simulink model "omnirover3wd_multibody"  (R2026a)
settings: Solver=ode15s  StopTime=simulationStopTime  MaxStep=0.01
PreLoadFcn:
  | run(fullfile(fileparts(get_param(bdroot,'FileName')),'parameters.m'))
InitFcn:
  | addpath(fileparts(get_param(bdroot,'FileName')))
values from neighbouring files (symbols this model uses):
  chassisMass = roverMass - 3*(servoMass + wheelMass)    (= 0.18)    [parameters.m]
  commandVxWorld = 0.12    [parameters.m]
  commandVyWorld = 0.06    [parameters.m]
  commandYawRateWorld = 0.35    [parameters.m]
  floorDeflectionFilterTime = 2e-3    (= 0.002)    [parameters.m]
  floorLateralFriction = 0.0    (= 0)    [parameters.m]
  floorLongitudinalDynamicFriction = 0.65    [parameters.m]
  floorNominalDeflection = floorNominalLoadPerWheel/floorNormalStiffness    [parameters.m]
  floorNormalDamping = 450    [parameters.m]
  floorNormalStiffness = 1.5e5    (= 150000)    [parameters.m]
  servoMass = 0.055    [parameters.m]
  servoMaxSpeed = 62 * 2*pi / 60    (= 6.49262481742)    [parameters.m]
  wheelAngles = deg2rad([0 120 240])    [parameters.m]    (also in test_kinematics.m)
  wheelCenterRadius = roverDiameter/2 - wheelRadius    (= 0.056)    [parameters.m]    (also in test_kinematics.m)
  wheelForceLimit = servoMaxTorque / wheelRadius    (= 53.1193541667)    [parameters.m]
  wheelMass = 0.039    [parameters.m]
  wheelRadius = 0.024    [parameters.m]    (also in test_kinematics.m)
  wheelSpeedGain = -25    [parameters.m]
undefined symbols (not defined in the file or in its folder): omni3wdInverseKinematics, X, Y, Z
libraries: sm_lib x21, nesl_utility x19, sl_discontinuities x3
settings Model: Creator=cafdr  LastModifiedBy=cafdr

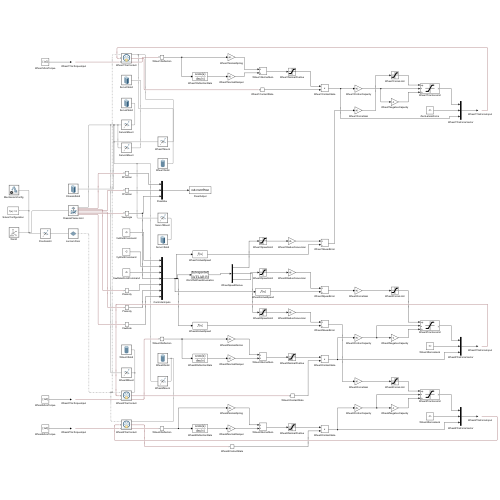
[thumbnail: Simulink's stored preview of the top-level diagram]
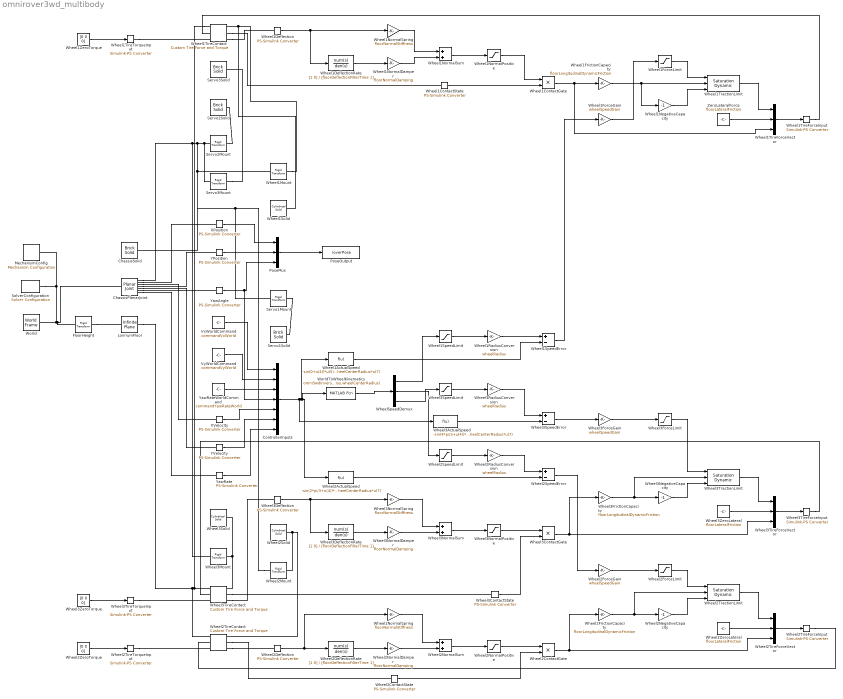
== system omnirover3wd_multibody ==
  ChassisPlanarJoint : sm_lib/Joints/Planar Joint  JointMode=Normal  CompositeWrenchDir=FollowerOnBase  CompositeWrenchFrame=BaseFrame  SenseConstraintForce=off  SenseConstraintTorque=off  SenseTotalForce=off  SenseTotalTorque=off  PxPositionTargetSpecify=off  PxPositionTargetPriority=High  PxPositionTargetValue=0  PxPositionTargetValueUnits=m  PxVelocityTargetSpecify=off  PxVelocityTargetPriority=High  PxVelocityTargetValue=0  PxVelocityTargetValueUnits=m/s  PxEquilibriumPosition=0  PxEquilibriumPositionUnits=m  PxSpringStiffness=0  PxSpringStiffnessUnits=N/m  PxDampingCoefficient=0  PxDampingCoefficientUnits=N/(m/s)  PxLowerLimitSpecify=off  PxLowerLimitBound=-1  PxLowerLimitBoundUnits=m  PxLowerLimitStiffness=1e6  PxLowerLimitStiffnessUnits=N/m  PxLowerLimitDamping=1e3  PxLowerLimitDampingUnits=N/(m/s)  PxLowerLimitTransitionRegionWidth=1e-4  PxLowerLimitTransitionRegionWidthUnits=m  PxUpperLimitSpecify=off  PxUpperLimitBound=1  PxUpperLimitBoundUnits=m  PxUpperLimitStiffness=1e6  PxUpperLimitStiffnessUnits=N/m  PxUpperLimitDamping=1e3  PxUpperLimitDampingUnits=N/(m/s)  PxUpperLimitTransitionRegionWidth=1e-4  PxUpperLimitTransitionRegionWidthUnits=m  PxTorqueActuationMode=NoTorque  PxMotionActuationMode=ComputedMotion  PxSensePosition=on  PxSenseVelocity=on  PxSenseAcceleration=off  PxSenseTorqueForce=off  PxSenseLowerLimitTorqueForce=off  PxSenseUpperLimitTorqueForce=off  PyPositionTargetSpecify=off  PyPositionTargetPriority=High  PyPositionTargetValue=0  PyPositionTargetValueUnits=m  PyVelocityTargetSpecify=off  PyVelocityTargetPriority=High  PyVelocityTargetValue=0  PyVelocityTargetValueUnits=m/s  PyEquilibriumPosition=0  PyEquilibriumPositionUnits=m  PySpringStiffness=0  PySpringStiffnessUnits=N/m  PyDampingCoefficient=0  PyDampingCoefficientUnits=N/(m/s)  PyLowerLimitSpecify=off  PyLowerLimitBound=-1  PyLowerLimitBoundUnits=m  PyLowerLimitStiffness=1e6  PyLowerLimitStiffnessUnits=N/m  PyLowerLimitDamping=1e3  PyLowerLimitDampingUnits=N/(m/s)  PyLowerLimitTransitionRegionWidth=1e-4  PyLowerLimitTransitionRegionWidthUnits=m  PyUpperLimitSpecify=off  PyUpperLimitBound=1  PyUpperLimitBoundUnits=m  PyUpperLimitStiffness=1e6  PyUpperLimitStiffnessUnits=N/m  PyUpperLimitDamping=1e3  PyUpperLimitDampingUnits=N/(m/s)  PyUpperLimitTransitionRegionWidth=1e-4  PyUpperLimitTransitionRegionWidthUnits=m  PyTorqueActuationMode=NoTorque  PyMotionActuationMode=ComputedMotion  PySensePosition=on  PySenseVelocity=on  PySenseAcceleration=off  PySenseTorqueForce=off  PySenseLowerLimitTorqueForce=off  PySenseUpperLimitTorqueForce=off  RzPositionTargetSpecify=off  RzPositionTargetPriority=High  RzPositionTargetValue=0  RzPositionTargetValueUnits=rad  RzVelocityTargetSpecify=off  RzVelocityTargetPriority=High  RzVelocityTargetValue=0  RzVelocityTargetValueUnits=rad/s  RzEquilibriumPosition=0  RzEquilibriumPositionUnits=deg  RzSpringStiffness=0  RzSpringStiffnessUnits=N*m/deg  RzDampingCoefficient=0  RzDampingCoefficientUnits=N*m/(deg/s)  RzLowerLimitSpecify=off  RzLowerLimitBound=-90  RzLowerLimitBoundUnits=deg  RzLowerLimitStiffness=1e4  RzLowerLimitStiffnessUnits=N*m/deg  RzLowerLimitDamping=10  RzLowerLimitDampingUnits=N*m/(deg/s)  RzLowerLimitTransitionRegionWidth=0.1  RzLowerLimitTransitionRegionWidthUnits=deg  RzUpperLimitSpecify=off  RzUpperLimitBound=90  RzUpperLimitBoundUnits=deg  RzUpperLimitStiffness=1e4  RzUpperLimitStiffnessUnits=N*m/deg  RzUpperLimitDamping=10  RzUpperLimitDampingUnits=N*m/(deg/s)  RzUpperLimitTransitionRegionWidth=0.1  RzUpperLimitTransitionRegionWidthUnits=deg  RzTorqueActuationMode=NoTorque  RzMotionActuationMode=ComputedMotion  RzSensePosition=on  RzSenseVelocity=on  RzSenseAcceleration=off  RzSenseTorqueForce=off  RzSenseLowerLimitTorqueForce=off  RzSenseUpperLimitTorqueForce=off
  ChassisSolid : sm_lib/Body Elements/Brick Solid  BrickDimensions=chassisDimensions  BrickDimensionsUnits=m  ExportEntireGeometry=off  InertiaType=CalculateFromGeometry  BasedOnType=Density  Density=1000  DensityUnits=kg/m^3  Mass=chassisMass  MassUnits=kg  CenterOfMass=[0 0 0]  CenterOfMassUnits=m  MomentsOfInertia=[1 1 1]  MomentsOfInertiaUnits=kg*m^2  ProductsOfInertia=[0 0 0]  ProductsOfInertiaUnits=kg*m^2  GraphicType=FromGeometry  MarkerShape=Sphere  MarkerSize=10  GraphicVisPropType=SimpleVisualProperties  GraphicDiffuseColor=[0.5 0.5 0.5]  GraphicOpacity=1  GraphicSpecularColor=[0.5 0.5 0.5 1.0]  GraphicAmbientColor=[0.15 0.15 0.15 1.0]  GraphicEmissiveColor=[0.0 0.0 0.0 1.0]  GraphicShininess=75  DoExposeReferenceFrame=on  SerializedFrames=<Frames/>
  ControllerInputs : Mux  Inputs=7
  FloorHeight : sm_lib/Frames and Transforms/Rigid Transform  RotationMethod=None  FollAlignAxisA=+X  BaseAlignAxisA=+Y  FollAlignAxisB=+Y  BaseAlignAxisB=+Z  RotationStandardAxis=+Z  RotationAngle=0  RotationAngleUnits=deg  RotationArbitraryAxis=[0 0 1]  RotationSequenceAxes=FollowerAxes  RotationSequence=XYX  RotationSequenceAngles=[0 0 0]  RotationSequenceAnglesUnits=deg  RotationMatrix=[1 0 0;0 1 0;0 0 1]  Quaternion=[1 0 0 0]  TranslationMethod=Cartesian  TranslationCartesianOffset=[0 0 -wheelRadius+floorNominalDeflection]  TranslationCartesianOffsetUnits=m  TranslationStandardAxis=+Z  TranslationStandardOffset=0  TranslationStandardOffsetUnits=m  TranslationROffset=0  TranslationROffsetUnits=m  TranslationThetaOffset=0  TranslationThetaOffsetUnits=deg  TranslationZOffset=0  TranslationZOffsetUnits=m
  LonriumFloor : sm_lib/Curves and Surfaces/Infinite Plane  GraphicType=Rectangle  GraphicPlaneWidth=2  GraphicPlaneWidthUnits=m  GraphicPlaneHeight=2  GraphicPlaneHeightUnits=m  GraphicVisPropType=SimpleVisualProperties  GraphicDiffuseColor=[0.55 0.58 0.62]  GraphicOpacity=1  GraphicSpecularColor=[0.5 0.5 0.5 1.0]  GraphicAmbientColor=[0.15 0.15 0.15 1.0]  GraphicEmissiveColor=[0.0 0.0 0.0 1.0]  GraphicShininess=75
  MechanismConfig : sm_lib/Utilities/Mechanism Configuration  UniformGravity=Constant  GravityVector=[0 0 -9.80665]  GravityVectorUnits=m/s^2  LinearizationDelta=0.001  JointModeTransitionNonlinearIterations=2
  PoseMux : Mux  Inputs=3
  PoseOutput : ToWorkspace  VariableName=roverPose  SaveFormat=Timeseries  SampleTime=-1
  Servo1Mount : sm_lib/Frames and Transforms/Rigid Transform  RotationMethod=RotationSequence  FollAlignAxisA=+X  BaseAlignAxisA=+Y  FollAlignAxisB=+Y  BaseAlignAxisB=+Z  RotationStandardAxis=+Z  RotationAngle=0  RotationAngleUnits=deg  RotationArbitraryAxis=[0 0 1]  RotationSequenceAxes=FollowerAxes  RotationSequence=ZYX  RotationSequenceAngles=[0 0 0]  RotationSequenceAnglesUnits=deg  RotationMatrix=[1 0 0;0 1 0;0 0 1]  Quaternion=[1 0 0 0]  TranslationMethod=Cartesian  TranslationCartesianOffset=(wheelCenterRadius-0.025)*[1 0 0]  TranslationCartesianOffsetUnits=m  TranslationStandardAxis=+Z  TranslationStandardOffset=0  TranslationStandardOffsetUnits=m  TranslationROffset=0  TranslationROffsetUnits=m  TranslationThetaOffset=0  TranslationThetaOffsetUnits=deg  TranslationZOffset=0  TranslationZOffsetUnits=m
  Servo1Solid : sm_lib/Body Elements/Brick Solid  BrickDimensions=servoDimensions  BrickDimensionsUnits=m  ExportEntireGeometry=off  InertiaType=CalculateFromGeometry  BasedOnType=Density  Density=1000  DensityUnits=kg/m^3  Mass=servoMass  MassUnits=kg  CenterOfMass=[0 0 0]  CenterOfMassUnits=m  MomentsOfInertia=[1 1 1]  MomentsOfInertiaUnits=kg*m^2  ProductsOfInertia=[0 0 0]  ProductsOfInertiaUnits=kg*m^2  GraphicType=FromGeometry  MarkerShape=Sphere  MarkerSize=10  GraphicVisPropType=SimpleVisualProperties  GraphicDiffuseColor=[0.5 0.5 0.5]  GraphicOpacity=1  GraphicSpecularColor=[0.5 0.5 0.5 1.0]  GraphicAmbientColor=[0.15 0.15 0.15 1.0]  GraphicEmissiveColor=[0.0 0.0 0.0 1.0]  GraphicShininess=75  DoExposeReferenceFrame=on  SerializedFrames=<Frames/>
  Servo2Mount : sm_lib/Frames and Transforms/Rigid Transform  RotationMethod=RotationSequence  FollAlignAxisA=+X  BaseAlignAxisA=+Y  FollAlignAxisB=+Y  BaseAlignAxisB=+Z  RotationStandardAxis=+Z  RotationAngle=0  RotationAngleUnits=deg  RotationArbitraryAxis=[0 0 1]  RotationSequenceAxes=FollowerAxes  RotationSequence=ZYX  RotationSequenceAngles=[120 0 0]  RotationSequenceAnglesUnits=deg  RotationMatrix=[1 0 0;0 1 0;0 0 1]  Quaternion=[1 0 0 0]  TranslationMethod=Cartesian  TranslationCartesianOffset=(wheelCenterRadius-0.025)*[cos(2*pi/3) sin(2*pi/3) 0]  TranslationCartesianOffsetUnits=m  TranslationStandardAxis=+Z  TranslationStandardOffset=0  TranslationStandardOffsetUnits=m  TranslationROffset=0  TranslationROffsetUnits=m  TranslationThetaOffset=0  TranslationThetaOffsetUnits=deg  TranslationZOffset=0  TranslationZOffsetUnits=m
  Servo2Solid : sm_lib/Body Elements/Brick Solid  BrickDimensions=servoDimensions  BrickDimensionsUnits=m  ExportEntireGeometry=off  InertiaType=CalculateFromGeometry  BasedOnType=Density  Density=1000  DensityUnits=kg/m^3  Mass=servoMass  MassUnits=kg  CenterOfMass=[0 0 0]  CenterOfMassUnits=m  MomentsOfInertia=[1 1 1]  MomentsOfInertiaUnits=kg*m^2  ProductsOfInertia=[0 0 0]  ProductsOfInertiaUnits=kg*m^2  GraphicType=FromGeometry  MarkerShape=Sphere  MarkerSize=10  GraphicVisPropType=SimpleVisualProperties  GraphicDiffuseColor=[0.5 0.5 0.5]  GraphicOpacity=1  GraphicSpecularColor=[0.5 0.5 0.5 1.0]  GraphicAmbientColor=[0.15 0.15 0.15 1.0]  GraphicEmissiveColor=[0.0 0.0 0.0 1.0]  GraphicShininess=75  DoExposeReferenceFrame=on  SerializedFrames=<Frames/>
  Servo3Mount : sm_lib/Frames and Transforms/Rigid Transform  RotationMethod=RotationSequence  FollAlignAxisA=+X  BaseAlignAxisA=+Y  FollAlignAxisB=+Y  BaseAlignAxisB=+Z  RotationStandardAxis=+Z  RotationAngle=0  RotationAngleUnits=deg  RotationArbitraryAxis=[0 0 1]  RotationSequenceAxes=FollowerAxes  RotationSequence=ZYX  RotationSequenceAngles=[240 0 0]  RotationSequenceAnglesUnits=deg  RotationMatrix=[1 0 0;0 1 0;0 0 1]  Quaternion=[1 0 0 0]  TranslationMethod=Cartesian  TranslationCartesianOffset=(wheelCenterRadius-0.025)*[cos(4*pi/3) sin(4*pi/3) 0]  TranslationCartesianOffsetUnits=m  TranslationStandardAxis=+Z  TranslationStandardOffset=0  TranslationStandardOffsetUnits=m  TranslationROffset=0  TranslationROffsetUnits=m  TranslationThetaOffset=0  TranslationThetaOffsetUnits=deg  TranslationZOffset=0  TranslationZOffsetUnits=m
  Servo3Solid : sm_lib/Body Elements/Brick Solid  BrickDimensions=servoDimensions  BrickDimensionsUnits=m  ExportEntireGeometry=off  InertiaType=CalculateFromGeometry  BasedOnType=Density  Density=1000  DensityUnits=kg/m^3  Mass=servoMass  MassUnits=kg  CenterOfMass=[0 0 0]  CenterOfMassUnits=m  MomentsOfInertia=[1 1 1]  MomentsOfInertiaUnits=kg*m^2  ProductsOfInertia=[0 0 0]  ProductsOfInertiaUnits=kg*m^2  GraphicType=FromGeometry  MarkerShape=Sphere  MarkerSize=10  GraphicVisPropType=SimpleVisualProperties  GraphicDiffuseColor=[0.5 0.5 0.5]  GraphicOpacity=1  GraphicSpecularColor=[0.5 0.5 0.5 1.0]  GraphicAmbientColor=[0.15 0.15 0.15 1.0]  GraphicEmissiveColor=[0.0 0.0 0.0 1.0]  GraphicShininess=75  DoExposeReferenceFrame=on  SerializedFrames=<Frames/>
  SolverConfiguration : nesl_utility/Solver Configuration  PhysicalDomain=network_engine_domain  SubClassName=solver  LeftPortType=input  RightPortType=generic  Tones=[]  Harmonics=[]  SimulateNoise=off  Profile=off  UseLocalSampling=off  EnableSwitchedLinearOptims=on  FrequencyDomain=off  UseCCode=off  RelTol=0.001  AbsTol=0.001  MinStep=1e-09  ToWorkspace=off  RevertToSquareIcSolve=off  NumHomotopyIterations=100  PhasorMode=off  PhasorModeNumHarmonics=1  ConsistencySolver=NEWTON_XTOL_AFTER_FTOL  CanonicalOrdering=CANONICAL  OptimizeIntermediates=OPTIMIZED  IndexReductionMethod=DerivativeReplacement  DoDC=off  ResidualTolerance=1e-09  ConsistencyTolSource=GLOBAL  ConsistencyAbsTol=0.001  ConsistencyRelTol=0.001  ConsistencyTolFactor=0.001  UseLocalSolver=off  LocalSolverChoice=NE_BACKWARD_EULER_ADVANCER  ResolveIndetEquations=on  FunctionEvalNumThread=1  LocalSolverSampleTime=0.001  DoFixedCost=off  MaxNonlinIter=3  MaxModeIter=2  ComputeImpulses=off  ImpulseIterations=2  LinearAlgebra=auto  LinearAlgebraNumThread=0  EquationFormulation=NE_TIME_EF  DelaysMemoryBudget=1024  AutomaticFiltering=on  FilteringTimeConstant=0.001  PartitionStorageMethod=AS_NEEDED  PartitionMemoryBudget=1024  PartitionMethod=ROBUST  MultibodyUseLocalSolver=off  MultibodyLocalSolverChoice=ODE1  MultibodyLocalSolverSampleTime=0.001
  VxWorldCommand : Constant  Value=commandVxWorld
  VyWorldCommand : Constant  Value=commandVyWorld
  Wheel1ActualSpeed : Fcn  Expr=-sin(0+u(4))*u(5)+cos(0+u(4))*u(6)+wheelCenterRadius*u(7)
  Wheel1ContactGate : Product  Inputs=**
  Wheel1ContactState : nesl_utility/PS-Simulink Converter  PhysicalDomain=network_engine_domain  SubClassName=ps_output  LeftPortType=input  RightPortType=output  PseudoPeriodic=off  Frequencies=[]  VectorFormat=inherit  Unit=1  AffineConversion=off
  Wheel1Deflection : nesl_utility/PS-Simulink Converter  PhysicalDomain=network_engine_domain  SubClassName=ps_output  LeftPortType=input  RightPortType=output  PseudoPeriodic=off  Frequencies=[]  VectorFormat=inherit  Unit=m  AffineConversion=off
  Wheel1DeflectionRate : TransferFcn  Numerator=[1 0]  Denominator=[floorDeflectionFilterTime 1]
  Wheel1ForceGain : Gain  Gain=wheelSpeedGain
  Wheel1ForceLimit : Saturate  UpperLimit=wheelForceLimit  LowerLimit=-wheelForceLimit
  Wheel1FrictionCapacity : Gain  Gain=floorLongitudinalDynamicFriction
  Wheel1Mount : sm_lib/Frames and Transforms/Rigid Transform  RotationMethod=RotationSequence  FollAlignAxisA=+X  BaseAlignAxisA=+Y  FollAlignAxisB=+Y  BaseAlignAxisB=+Z  RotationStandardAxis=+Z  RotationAngle=0  RotationAngleUnits=deg  RotationArbitraryAxis=[0 0 1]  RotationSequenceAxes=FollowerAxes  RotationSequence=ZYX  RotationSequenceAngles=[0 90 0]  RotationSequenceAnglesUnits=deg  RotationMatrix=[1 0 0;0 1 0;0 0 1]  Quaternion=[1 0 0 0]  TranslationMethod=Cartesian  TranslationCartesianOffset=[wheelCenterRadius 0 0]  TranslationCartesianOffsetUnits=m  TranslationStandardAxis=+Z  TranslationStandardOffset=0  TranslationStandardOffsetUnits=m  TranslationROffset=0  TranslationROffsetUnits=m  TranslationThetaOffset=0  TranslationThetaOffsetUnits=deg  TranslationZOffset=0  TranslationZOffsetUnits=m
  Wheel1NegativeCapacity : Gain  Gain=-1
  Wheel1NormalDamper : Gain  Gain=floorNormalDamping
  Wheel1NormalPositive : Saturate  UpperLimit=inf  LowerLimit=0
  Wheel1NormalSpring : Gain  Gain=floorNormalStiffness
  Wheel1NormalSum : Sum
  Wheel1RadiusConversion : Gain  Gain=wheelRadius
  Wheel1Solid : sm_lib/Body Elements/Cylindrical Solid  CylinderRadius=wheelRadius  CylinderRadiusUnits=m  CylinderLength=wheelWidth  CylinderLengthUnits=m  ExportEntireGeometry=off  InertiaType=CalculateFromGeometry  BasedOnType=Density  Density=1000  DensityUnits=kg/m^3  Mass=wheelMass  MassUnits=kg  CenterOfMass=[0 0 0]  CenterOfMassUnits=m  MomentsOfInertia=[1 1 1]  MomentsOfInertiaUnits=kg*m^2  ProductsOfInertia=[0 0 0]  ProductsOfInertiaUnits=kg*m^2  GraphicType=FromGeometry  MarkerShape=Sphere  MarkerSize=10  GraphicVisPropType=SimpleVisualProperties  GraphicDiffuseColor=[0.5 0.5 0.5]  GraphicOpacity=1  GraphicSpecularColor=[0.5 0.5 0.5 1.0]  GraphicAmbientColor=[0.15 0.15 0.15 1.0]  GraphicEmissiveColor=[0.0 0.0 0.0 1.0]  GraphicShininess=75  DoExposeReferenceFrame=on  SerializedFrames=<Frames/>
  Wheel1SpeedError : Sum  Inputs=+-
  Wheel1SpeedLimit : Saturate  UpperLimit=servoMaxSpeed  LowerLimit=-servoMaxSpeed
  Wheel1TireContact : sm_lib/Forces and Torques/Custom Tire Force and Torque  TireRadius=wheelRadius  TireRadiusUnits=m  ContactFrameMethod=ClosestPoint  SenseContactSignal=on  SenseRelativeLongitudinalVelocity=off  SenseRelativeLateralVelocity=off  SenseYawVelocity=off  SenseCamberAngle=off  SenseCamberVelocity=off  SenseSpinVelocity=off  SenseLoadedRadius=off  SenseRadialDeflection=on  SenseContactBaseRotation=off  SenseContactBaseTranslation=off  SenseContactFollowerRotation=off  SenseContactFollowerTranslation=off
  Wheel1TireForceInput : nesl_utility/Simulink-PS Converter  PhysicalDomain=network_engine_domain  SubClassName=ps_input  LeftPortType=input  RightPortType=output  PseudoPeriodic=off  Frequencies=[]  NoiseDistribution=none  NoiseParameters=[]  Unit=N  AffineConversion=off  FilteringAndDerivatives=provide  SimscapeFilterOrder=1  InputFilterTimeConstant=0.001  UdotUserProvided=0
  Wheel1TireForceVector : Mux  Inputs=3
  Wheel1TireTorqueInput : nesl_utility/Simulink-PS Converter  PhysicalDomain=network_engine_domain  SubClassName=ps_input  LeftPortType=input  RightPortType=output  PseudoPeriodic=off  Frequencies=[]  NoiseDistribution=none  NoiseParameters=[]  Unit=N*m  AffineConversion=off  FilteringAndDerivatives=provide  SimscapeFilterOrder=1  InputFilterTimeConstant=0.001  UdotUserProvided=0
  Wheel1TractionLimit : sl_discontinuities/Saturation Dynamic  OutMin=[]  OutMax=[]  OutDataTypeStr=Inherit: Same as second input  OutDataType=fixdt(1, 16)  OutScaling=2^-10  DoSatur=off
      settings: LibrarySourceBlock=|
      | simulink/Discontinuities/Saturation
      | Dynamic
  Wheel1ZeroTorque : Constant  Value=[0 0 0]
  Wheel2ActualSpeed : Fcn  Expr=-sin(2*pi/3+u(4))*u(5)+cos(2*pi/3+u(4))*u(6)+wheelCenterRadius*u(7)
  Wheel2ContactGate : Product  Inputs=**
  Wheel2ContactState : nesl_utility/PS-Simulink Converter  PhysicalDomain=network_engine_domain  SubClassName=ps_output  LeftPortType=input  RightPortType=output  PseudoPeriodic=off  Frequencies=[]  VectorFormat=inherit  Unit=1  AffineConversion=off
  Wheel2Deflection : nesl_utility/PS-Simulink Converter  PhysicalDomain=network_engine_domain  SubClassName=ps_output  LeftPortType=input  RightPortType=output  PseudoPeriodic=off  Frequencies=[]  VectorFormat=inherit  Unit=m  AffineConversion=off
  Wheel2DeflectionRate : TransferFcn  Numerator=[1 0]  Denominator=[floorDeflectionFilterTime 1]
  Wheel2ForceGain : Gain  Gain=wheelSpeedGain
  Wheel2ForceLimit : Saturate  UpperLimit=wheelForceLimit  LowerLimit=-wheelForceLimit
  Wheel2FrictionCapacity : Gain  Gain=floorLongitudinalDynamicFriction
  Wheel2Mount : sm_lib/Frames and Transforms/Rigid Transform  RotationMethod=RotationSequence  FollAlignAxisA=+X  BaseAlignAxisA=+Y  FollAlignAxisB=+Y  BaseAlignAxisB=+Z  RotationStandardAxis=+Z  RotationAngle=0  RotationAngleUnits=deg  RotationArbitraryAxis=[0 0 1]  RotationSequenceAxes=FollowerAxes  RotationSequence=ZYX  RotationSequenceAngles=[120 90 0]  RotationSequenceAnglesUnits=deg  RotationMatrix=[1 0 0;0 1 0;0 0 1]  Quaternion=[1 0 0 0]  TranslationMethod=Cartesian  TranslationCartesianOffset=wheelCenterRadius*[cos(2*pi/3) sin(2*pi/3) 0]  TranslationCartesianOffsetUnits=m  TranslationStandardAxis=+Z  TranslationStandardOffset=0  TranslationStandardOffsetUnits=m  TranslationROffset=0  TranslationROffsetUnits=m  TranslationThetaOffset=0  TranslationThetaOffsetUnits=deg  TranslationZOffset=0  TranslationZOffsetUnits=m
  Wheel2NegativeCapacity : Gain  Gain=-1
  Wheel2NormalDamper : Gain  Gain=floorNormalDamping
  Wheel2NormalPositive : Saturate  UpperLimit=inf  LowerLimit=0
  Wheel2NormalSpring : Gain  Gain=floorNormalStiffness
  Wheel2NormalSum : Sum
  Wheel2RadiusConversion : Gain  Gain=wheelRadius
  Wheel2Solid : sm_lib/Body Elements/Cylindrical Solid  CylinderRadius=wheelRadius  CylinderRadiusUnits=m  CylinderLength=wheelWidth  CylinderLengthUnits=m  ExportEntireGeometry=off  InertiaType=CalculateFromGeometry  BasedOnType=Density  Density=1000  DensityUnits=kg/m^3  Mass=wheelMass  MassUnits=kg  CenterOfMass=[0 0 0]  CenterOfMassUnits=m  MomentsOfInertia=[1 1 1]  MomentsOfInertiaUnits=kg*m^2  ProductsOfInertia=[0 0 0]  ProductsOfInertiaUnits=kg*m^2  GraphicType=FromGeometry  MarkerShape=Sphere  MarkerSize=10  GraphicVisPropType=SimpleVisualProperties  GraphicDiffuseColor=[0.5 0.5 0.5]  GraphicOpacity=1  GraphicSpecularColor=[0.5 0.5 0.5 1.0]  GraphicAmbientColor=[0.15 0.15 0.15 1.0]  GraphicEmissiveColor=[0.0 0.0 0.0 1.0]  GraphicShininess=75  DoExposeReferenceFrame=on  SerializedFrames=<Frames/>
  Wheel2SpeedError : Sum  Inputs=+-
  Wheel2SpeedLimit : Saturate  UpperLimit=servoMaxSpeed  LowerLimit=-servoMaxSpeed
  Wheel2TireContact : sm_lib/Forces and Torques/Custom Tire Force and Torque  TireRadius=wheelRadius  TireRadiusUnits=m  ContactFrameMethod=ClosestPoint  SenseContactSignal=on  SenseRelativeLongitudinalVelocity=off  SenseRelativeLateralVelocity=off  SenseYawVelocity=off  SenseCamberAngle=off  SenseCamberVelocity=off  SenseSpinVelocity=off  SenseLoadedRadius=off  SenseRadialDeflection=on  SenseContactBaseRotation=off  SenseContactBaseTranslation=off  SenseContactFollowerRotation=off  SenseContactFollowerTranslation=off
  Wheel2TireForceInput : nesl_utility/Simulink-PS Converter  PhysicalDomain=network_engine_domain  SubClassName=ps_input  LeftPortType=input  RightPortType=output  PseudoPeriodic=off  Frequencies=[]  NoiseDistribution=none  NoiseParameters=[]  Unit=N  AffineConversion=off  FilteringAndDerivatives=provide  SimscapeFilterOrder=1  InputFilterTimeConstant=0.001  UdotUserProvided=0
  Wheel2TireForceVector : Mux  Inputs=3
  Wheel2TireTorqueInput : nesl_utility/Simulink-PS Converter  PhysicalDomain=network_engine_domain  SubClassName=ps_input  LeftPortType=input  RightPortType=output  PseudoPeriodic=off  Frequencies=[]  NoiseDistribution=none  NoiseParameters=[]  Unit=N*m  AffineConversion=off  FilteringAndDerivatives=provide  SimscapeFilterOrder=1  InputFilterTimeConstant=0.001  UdotUserProvided=0
  Wheel2TractionLimit : sl_discontinuities/Saturation Dynamic  OutMin=[]  OutMax=[]  OutDataTypeStr=Inherit: Same as second input  OutDataType=fixdt(1, 16)  OutScaling=2^-10  DoSatur=off
      settings: LibrarySourceBlock=|
      | simulink/Discontinuities/Saturation
      | Dynamic
  Wheel2ZeroLateral : Constant  Value=floorLateralFriction
  Wheel2ZeroTorque : Constant  Value=[0 0 0]
  Wheel3ActualSpeed : Fcn  Expr=-sin(4*pi/3+u(4))*u(5)+cos(4*pi/3+u(4))*u(6)+wheelCenterRadius*u(7)
  Wheel3ContactGate : Product  Inputs=**
  Wheel3ContactState : nesl_utility/PS-Simulink Converter  PhysicalDomain=network_engine_domain  SubClassName=ps_output  LeftPortType=input  RightPortType=output  PseudoPeriodic=off  Frequencies=[]  VectorFormat=inherit  Unit=1  AffineConversion=off
  Wheel3Deflection : nesl_utility/PS-Simulink Converter  PhysicalDomain=network_engine_domain  SubClassName=ps_output  LeftPortType=input  RightPortType=output  PseudoPeriodic=off  Frequencies=[]  VectorFormat=inherit  Unit=m  AffineConversion=off
  Wheel3DeflectionRate : TransferFcn  Numerator=[1 0]  Denominator=[floorDeflectionFilterTime 1]
  Wheel3ForceGain : Gain  Gain=wheelSpeedGain
  Wheel3ForceLimit : Saturate  UpperLimit=wheelForceLimit  LowerLimit=-wheelForceLimit
  Wheel3FrictionCapacity : Gain  Gain=floorLongitudinalDynamicFriction
  Wheel3Mount : sm_lib/Frames and Transforms/Rigid Transform  RotationMethod=RotationSequence  FollAlignAxisA=+X  BaseAlignAxisA=+Y  FollAlignAxisB=+Y  BaseAlignAxisB=+Z  RotationStandardAxis=+Z  RotationAngle=0  RotationAngleUnits=deg  RotationArbitraryAxis=[0 0 1]  RotationSequenceAxes=FollowerAxes  RotationSequence=ZYX  RotationSequenceAngles=[240 90 0]  RotationSequenceAnglesUnits=deg  RotationMatrix=[1 0 0;0 1 0;0 0 1]  Quaternion=[1 0 0 0]  TranslationMethod=Cartesian  TranslationCartesianOffset=wheelCenterRadius*[cos(4*pi/3) sin(4*pi/3) 0]  TranslationCartesianOffsetUnits=m  TranslationStandardAxis=+Z  TranslationStandardOffset=0  TranslationStandardOffsetUnits=m  TranslationROffset=0  TranslationROffsetUnits=m  TranslationThetaOffset=0  TranslationThetaOffsetUnits=deg  TranslationZOffset=0  TranslationZOffsetUnits=m
  Wheel3NegativeCapacity : Gain  Gain=-1
  Wheel3NormalDamper : Gain  Gain=floorNormalDamping
  Wheel3NormalPositive : Saturate  UpperLimit=inf  LowerLimit=0
  Wheel3NormalSpring : Gain  Gain=floorNormalStiffness
  Wheel3NormalSum : Sum
  Wheel3RadiusConversion : Gain  Gain=wheelRadius
  Wheel3Solid : sm_lib/Body Elements/Cylindrical Solid  CylinderRadius=wheelRadius  CylinderRadiusUnits=m  CylinderLength=wheelWidth  CylinderLengthUnits=m  ExportEntireGeometry=off  InertiaType=CalculateFromGeometry  BasedOnType=Density  Density=1000  DensityUnits=kg/m^3  Mass=wheelMass  MassUnits=kg  CenterOfMass=[0 0 0]  CenterOfMassUnits=m  MomentsOfInertia=[1 1 1]  MomentsOfInertiaUnits=kg*m^2  ProductsOfInertia=[0 0 0]  ProductsOfInertiaUnits=kg*m^2  GraphicType=FromGeometry  MarkerShape=Sphere  MarkerSize=10  GraphicVisPropType=SimpleVisualProperties  GraphicDiffuseColor=[0.5 0.5 0.5]  GraphicOpacity=1  GraphicSpecularColor=[0.5 0.5 0.5 1.0]  GraphicAmbientColor=[0.15 0.15 0.15 1.0]  GraphicEmissiveColor=[0.0 0.0 0.0 1.0]  GraphicShininess=75  DoExposeReferenceFrame=on  SerializedFrames=<Frames/>
  Wheel3SpeedError : Sum  Inputs=+-
  Wheel3SpeedLimit : Saturate  UpperLimit=servoMaxSpeed  LowerLimit=-servoMaxSpeed
  Wheel3TireContact : sm_lib/Forces and Torques/Custom Tire Force and Torque  TireRadius=wheelRadius  TireRadiusUnits=m  ContactFrameMethod=ClosestPoint  SenseContactSignal=on  SenseRelativeLongitudinalVelocity=off  SenseRelativeLateralVelocity=off  SenseYawVelocity=off  SenseCamberAngle=off  SenseCamberVelocity=off  SenseSpinVelocity=off  SenseLoadedRadius=off  SenseRadialDeflection=on  SenseContactBaseRotation=off  SenseContactBaseTranslation=off  SenseContactFollowerRotation=off  SenseContactFollowerTranslation=off
  Wheel3TireForceInput : nesl_utility/Simulink-PS Converter  PhysicalDomain=network_engine_domain  SubClassName=ps_input  LeftPortType=input  RightPortType=output  PseudoPeriodic=off  Frequencies=[]  NoiseDistribution=none  NoiseParameters=[]  Unit=N  AffineConversion=off  FilteringAndDerivatives=provide  SimscapeFilterOrder=1  InputFilterTimeConstant=0.001  UdotUserProvided=0
  Wheel3TireForceVector : Mux  Inputs=3
  Wheel3TireTorqueInput : nesl_utility/Simulink-PS Converter  PhysicalDomain=network_engine_domain  SubClassName=ps_input  LeftPortType=input  RightPortType=output  PseudoPeriodic=off  Frequencies=[]  NoiseDistribution=none  NoiseParameters=[]  Unit=N*m  AffineConversion=off  FilteringAndDerivatives=provide  SimscapeFilterOrder=1  InputFilterTimeConstant=0.001  UdotUserProvided=0
  Wheel3TractionLimit : sl_discontinuities/Saturation Dynamic  OutMin=[]  OutMax=[]  OutDataTypeStr=Inherit: Same as second input  OutDataType=fixdt(1, 16)  OutScaling=2^-10  DoSatur=off
      settings: LibrarySourceBlock=|
      | simulink/Discontinuities/Saturation
      | Dynamic
  Wheel3ZeroLateral : Constant  Value=floorLateralFriction
  Wheel3ZeroTorque : Constant  Value=[0 0 0]
  WheelSpeedDemux : Demux  Outputs=3
  World : sm_lib/Frames and Transforms/World Frame
  WorldToWheelKinematics : MATLABFcn  MATLABFcn=omni3wdInverseKinematics(u(1:3),u(4),wheelAngles,wheelRadius,wheelCenterRadius)  OutputDimensions=3
  XPosition : nesl_utility/PS-Simulink Converter  PhysicalDomain=network_engine_domain  SubClassName=ps_output  LeftPortType=input  RightPortType=output  PseudoPeriodic=off  Frequencies=[]  VectorFormat=inherit  Unit=m  AffineConversion=off
  XVelocity : nesl_utility/PS-Simulink Converter  PhysicalDomain=network_engine_domain  SubClassName=ps_output  LeftPortType=input  RightPortType=output  PseudoPeriodic=off  Frequencies=[]  VectorFormat=inherit  Unit=m/s  AffineConversion=off
  YPosition : nesl_utility/PS-Simulink Converter  PhysicalDomain=network_engine_domain  SubClassName=ps_output  LeftPortType=input  RightPortType=output  PseudoPeriodic=off  Frequencies=[]  VectorFormat=inherit  Unit=m  AffineConversion=off
  YVelocity : nesl_utility/PS-Simulink Converter  PhysicalDomain=network_engine_domain  SubClassName=ps_output  LeftPortType=input  RightPortType=output  PseudoPeriodic=off  Frequencies=[]  VectorFormat=inherit  Unit=m/s  AffineConversion=off
  YawAngle : nesl_utility/PS-Simulink Converter  PhysicalDomain=network_engine_domain  SubClassName=ps_output  LeftPortType=input  RightPortType=output  PseudoPeriodic=off  Frequencies=[]  VectorFormat=inherit  Unit=rad  AffineConversion=off
  YawRate : nesl_utility/PS-Simulink Converter  PhysicalDomain=network_engine_domain  SubClassName=ps_output  LeftPortType=input  RightPortType=output  PseudoPeriodic=off  Frequencies=[]  VectorFormat=inherit  Unit=rad/s  AffineConversion=off
  YawRateWorldCommand : Constant  Value=commandYawRateWorld
  ZeroLateralForce : Constant  Value=floorLateralFriction
  wires:
  Wheel3RadiusConversion/1 -> Wheel3SpeedError/1
  Wheel3SpeedLimit/1 -> Wheel3RadiusConversion/1
  Wheel2RadiusConversion/1 -> Wheel2SpeedError/1
  Wheel2SpeedLimit/1 -> Wheel2RadiusConversion/1
  Wheel1RadiusConversion/1 -> Wheel1SpeedError/1
  Wheel1SpeedLimit/1 -> Wheel1RadiusConversion/1
  WheelSpeedDemux/3 -> Wheel3SpeedLimit/1
  WheelSpeedDemux/2 -> Wheel2SpeedLimit/1
  WheelSpeedDemux/1 -> Wheel1SpeedLimit/1
  WorldToWheelKinematics/1 -> WheelSpeedDemux/1
  Wheel1ZeroTorque/1 -> Wheel1TireTorqueInput/1
  Wheel1TireForceVector/1 -> Wheel1TireForceInput/1
  ZeroLateralForce/1 -> Wheel1TireForceVector/2
  Wheel1ContactGate/1 -> Wheel1FrictionCapacity/1, Wheel1TireForceVector/3
  Wheel1ContactState/1 -> Wheel1ContactGate/2
  Wheel1NormalPositive/1 -> Wheel1ContactGate/1
  Wheel1NormalSum/1 -> Wheel1NormalPositive/1
  Wheel1NormalDamper/1 -> Wheel1NormalSum/2
  Wheel1NormalSpring/1 -> Wheel1NormalSum/1
  Wheel1DeflectionRate/1 -> Wheel1NormalDamper/1
  Wheel1Deflection/1 -> Wheel1NormalSpring/1, Wheel1DeflectionRate/1
  Wheel3SpeedError/1 -> Wheel3ForceGain/1
  Wheel3ActualSpeed/1 -> Wheel3SpeedError/2
  Wheel2SpeedError/1 -> Wheel2ForceGain/1
  Wheel2ActualSpeed/1 -> Wheel2SpeedError/2
  Wheel1SpeedError/1 -> Wheel1ForceGain/1
  Wheel1ActualSpeed/1 -> Wheel1SpeedError/2
  VxWorldCommand/1 -> ControllerInputs/1
  VyWorldCommand/1 -> ControllerInputs/2
  YawRateWorldCommand/1 -> ControllerInputs/3
  YawAngle/1 -> ControllerInputs/4, PoseMux/3
  XVelocity/1 -> ControllerInputs/5
  YVelocity/1 -> ControllerInputs/6
  YawRate/1 -> ControllerInputs/7
  ControllerInputs/1 -> Wheel2ActualSpeed/1, WorldToWheelKinematics/1, Wheel1ActualSpeed/1, Wheel3ActualSpeed/1
  XPosition/1 -> PoseMux/1
  YPosition/1 -> PoseMux/2
  PoseMux/1 -> PoseOutput/1
  Wheel1ForceGain/1 -> Wheel1ForceLimit/1
  Wheel2ForceGain/1 -> Wheel2ForceLimit/1
  Wheel3ForceGain/1 -> Wheel3ForceLimit/1
  Wheel2Deflection/1 -> Wheel2DeflectionRate/1, Wheel2NormalSpring/1
  Wheel2DeflectionRate/1 -> Wheel2NormalDamper/1
  Wheel2NormalSpring/1 -> Wheel2NormalSum/1
  Wheel2NormalDamper/1 -> Wheel2NormalSum/2
  Wheel2NormalSum/1 -> Wheel2NormalPositive/1
  Wheel2NormalPositive/1 -> Wheel2ContactGate/1
  Wheel2ContactState/1 -> Wheel2ContactGate/2
  Wheel2ContactGate/1 -> Wheel2TireForceVector/3, Wheel2FrictionCapacity/1
  Wheel2ZeroLateral/1 -> Wheel2TireForceVector/2
  Wheel2TireForceVector/1 -> Wheel2TireForceInput/1
  Wheel2ZeroTorque/1 -> Wheel2TireTorqueInput/1
  Wheel3Deflection/1 -> Wheel3DeflectionRate/1, Wheel3NormalSpring/1
  Wheel3DeflectionRate/1 -> Wheel3NormalDamper/1
  Wheel3NormalSpring/1 -> Wheel3NormalSum/1
  Wheel3NormalDamper/1 -> Wheel3NormalSum/2
  Wheel3NormalSum/1 -> Wheel3NormalPositive/1
  Wheel3NormalPositive/1 -> Wheel3ContactGate/1
  Wheel3ContactState/1 -> Wheel3ContactGate/2
  Wheel3ContactGate/1 -> Wheel3TireForceVector/3, Wheel3FrictionCapacity/1
  Wheel3ZeroLateral/1 -> Wheel3TireForceVector/2
  Wheel3TireForceVector/1 -> Wheel3TireForceInput/1
  Wheel3ZeroTorque/1 -> Wheel3TireTorqueInput/1
  Wheel1ForceLimit/1 -> Wheel1TractionLimit/1
  Wheel1FrictionCapacity/1 -> Wheel1NegativeCapacity/1, Wheel1TractionLimit/2
  Wheel1NegativeCapacity/1 -> Wheel1TractionLimit/3
  Wheel1TractionLimit/1 -> Wheel1TireForceVector/1
  Wheel2ForceLimit/1 -> Wheel2TractionLimit/1
  Wheel2FrictionCapacity/1 -> Wheel2NegativeCapacity/1, Wheel2TractionLimit/2
  Wheel2NegativeCapacity/1 -> Wheel2TractionLimit/3
  Wheel2TractionLimit/1 -> Wheel2TireForceVector/1
  Wheel3ForceLimit/1 -> Wheel3TractionLimit/1
  Wheel3FrictionCapacity/1 -> Wheel3NegativeCapacity/1, Wheel3TractionLimit/2
  Wheel3NegativeCapacity/1 -> Wheel3TractionLimit/3
  Wheel3TractionLimit/1 -> Wheel3TireForceVector/1
  connections:
  Wheel1TireTorqueInput/RConn1 -- Wheel1TireContact/LConn3
  Wheel1TireForceInput/RConn1 -- Wheel1TireContact/LConn2
  Wheel1TireContact/RConn2 -- Wheel1ContactState/LConn1
  Wheel1TireContact/RConn3 -- Wheel1Deflection/LConn1
  Servo3Mount/RConn1 -- Servo3Solid/RConn1
  Servo2Mount/RConn1 -- Servo2Solid/RConn1
  Servo1Mount/RConn1 -- Servo1Solid/RConn1
  Wheel3Solid/RConn1 -- Wheel3TireContact/RConn1 -- Wheel3Mount/RConn1
  Wheel2TireContact/RConn1 -- Wheel2Mount/RConn1 -- Wheel2Solid/RConn1
  ChassisPlanarJoint/RConn7 -- YawRate/LConn1
  ChassisPlanarJoint/RConn6 -- YawAngle/LConn1
  ChassisPlanarJoint/RConn5 -- YVelocity/LConn1
  ChassisPlanarJoint/RConn4 -- YPosition/LConn1
  ChassisPlanarJoint/RConn3 -- XVelocity/LConn1
  ChassisPlanarJoint/RConn2 -- XPosition/LConn1
  Wheel2Mount/LConn1 -- ChassisPlanarJoint/RConn1 -- Wheel3Mount/LConn1 -- ChassisSolid/RConn1 -- Servo2Mount/LConn1 -- Servo3Mount/LConn1 -- Wheel1Mount/LConn1 -- Servo1Mount/LConn1
  MechanismConfig/RConn1 -- ChassisPlanarJoint/LConn1 -- FloorHeight/LConn1 -- World/RConn1 -- SolverConfiguration/RConn1
  Wheel1Solid/RConn1 -- Wheel1TireContact/RConn1 -- Wheel1Mount/RConn1
  FloorHeight/RConn1 -- LonriumFloor/LConn1
  Wheel1TireContact/LConn1 -- LonriumFloor/RConn1 -- Wheel2TireContact/LConn1 -- Wheel3TireContact/LConn1
  Wheel2TireContact/RConn3 -- Wheel2Deflection/LConn1
  Wheel2TireContact/RConn2 -- Wheel2ContactState/LConn1
  Wheel2TireForceInput/RConn1 -- Wheel2TireContact/LConn2
  Wheel2TireTorqueInput/RConn1 -- Wheel2TireContact/LConn3
  Wheel3TireContact/RConn3 -- Wheel3Deflection/LConn1
  Wheel3TireContact/RConn2 -- Wheel3ContactState/LConn1
  Wheel3TireForceInput/RConn1 -- Wheel3TireContact/LConn2
  Wheel3TireTorqueInput/RConn1 -- Wheel3TireContact/LConn3
